simulink model "bldc_sim_combined_2024"  (R2025a)
settings: Solver=VariableStepAuto  StartTime=0.0  StopTime=1.5  RelTol=1e-3
values from neighbouring files (symbols this model uses):
  phi_corr_LUT_param = Simulink.Parameter(phi_corr_LUT)    [lut_script.m]
undefined symbols (not defined in the file or in its folder): closed_loop, D_duty_cycle, D_m, DiscIntNeverNeededParam, hall_errors, I_duty_cycle, J_t, L_ss, lambda_m, P, P_duty_cycle, r_s, R_vs, T_m, theta_v, use_LUT, V_bus
libraries: spsMosfetLib x6, spsSeriesRLCBranchLib x4, spsVoltageMeasurementLib x3, spsControlledCurrentSourceLib x3, slpidlib x2, eeGeneralControl x1, simulink x1, embmathops x1, spsControlledVoltageSourceLib x1, spsPWMGeneratorDCDCLib x1, spsDCVoltageSourceLib x1, sps_lib x1
(part 2 of 2)

== matlab function bldc_sim_combined_2024/hall_filter/MATLAB Function2 ==
  data: timer input; w_hw output; w_hw_filt output; w_sw output; w_lut output; hw_trig input; sw_trig input; hall_state input; lut_vals input; debug_angle output
function [w_hw, w_hw_filt, w_sw, w_lut, debug_angle] = speed_estimators(timer, hw_trig, sw_trig, hall_state, lut_vals)

    persistent t_prev_hw t_prev_sw
    persistent w_hw_store w_hw_filt_store w_sw_store w_lut_store
    persistent prev_hall_state
    persistent prev_hw_trig prev_sw_trig 
    
    PI_over_3 = pi/3; 
    ALPHA = 0.05; 
    
    if isempty(t_prev_hw)
        t_prev_hw = double(timer);
        t_prev_sw = double(timer);
        w_hw_store = 0; w_hw_filt_store = 0; w_sw_store = 0; w_lut_store = 0;
        prev_hall_state = 1; 
        prev_hw_trig = 0; prev_sw_trig = 0;
    end
    
    % Edge Detection
    hw_trig_d = double(hw_trig);
    sw_trig_d = double(sw_trig);
    trig_hw_now = (hw_trig_d == 1) && (prev_hw_trig == 0);
    trig_sw_now = (sw_trig_d > 0) && (prev_sw_trig == 0);
    prev_hw_trig = hw_trig_d; prev_sw_trig = sw_trig_d;

    % DEBUGGING VARIABLE 
    debug_angle = 0.0; 

    % HARDWARE ISR (Raw Hall Changes) 
    if trig_hw_now
        dt_hw = double(timer) - t_prev_hw;
        
        if dt_hw > 1e-6
            % 1. Raw HW
            w_hw_store = PI_over_3 / dt_hw;
            
            % 2. Filtered
            w_hw_filt_store = (ALPHA * w_hw_store) + ((1 - ALPHA) * w_hw_filt_store);
            
            % 4. LUT Based
            % CRITICAL: We use 'prev_hall_state' because that is the state we just spent 'dt_hw' inside.
            idx = mod((prev_hall_state) + 1, 6);
            
            % SAFETY: Ensure index is 1..6
            if idx < 1; idx = 1; end; 
            if idx > 6; idx = 6; end;
            
            % Fetch angle
            actual_angle = double(lut_vals(idx));
            
            % Calculate Speed
            w_lut_store = actual_angle / dt_hw;
            
            % Debug output to check if we are grabbing the right values
            debug_angle = actual_angle;
            
            % Update History
            t_prev_hw = double(timer);
            prev_hall_state = double(hall_state); % Capture current state for NEXT time
        end
    end

    % SOFTWARE ISR 
    if trig_sw_now
        dt_sw = double(timer) - t_prev_sw;
        if dt_sw > 1e-6
            w_sw_store = PI_over_3 / dt_sw;
            t_prev_sw = double(timer);
        end
    end

    % Outputs
    w_hw = w_hw_store;
    w_hw_filt = w_hw_filt_store;
    w_sw = w_sw_store;
    w_lut = w_lut_store;
    
    % % If logic didn't run, output the last calculated angle
    % if debug_angle == 0.0
    %      % For now, 0 implies no update this step.
    % end
end

== matlab function bldc_sim_combined_2024/MATLAB Function ==
  data: H1 input; HALL_STATE output; H2 input; H3 input
function HALL_STATE = hall_to_statenum(H1,H2,H3)
HALL_STATE = 4*H1 + 2*H2 + H3;

== matlab function bldc_sim_combined_2024/hall_filter/First trigger initialization/MATLAB Function ==
  data: num input; interval output
function interval = num_to_interval(num)
DICT = [5,3,4,1,6,2];
interval = DICT(num);

== matlab function bldc_sim_combined_2024/MATLAB Function1 ==
  data: omega_r input; f_Hz output
function f_Hz = avg_freq_sim(omega_r)
f_Hz = avg_freq(omega_r);

== matlab function bldc_sim_combined_2024/hall_filter/MATLAB Function ==
  data: H1 input; HALL_STATE output; H2 input; H3 input
function HALL_STATE = hall_to_statenum(H1,H2,H3)
HALL_STATE = 4*H1 + 2*H2 + H3;
